simulink model "SB3_subsys_done"  (R2024b)
settings: Solver=FixedStepDiscrete  StartTime=0.0  StopTime=5  FixedStep=0.05  RelTol=1e-3
settings Model: Creator=admin  LastModifiedBy=admin

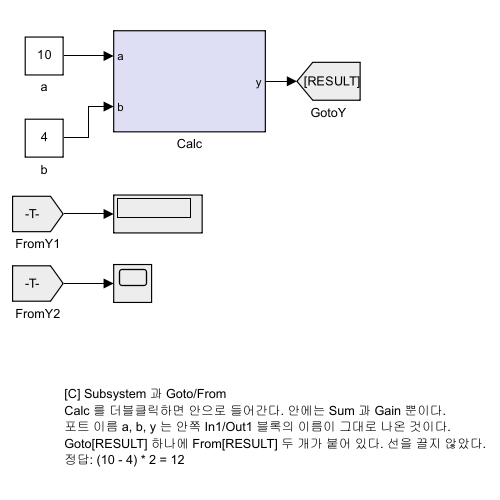
[thumbnail: Simulink's stored preview of the top-level diagram]
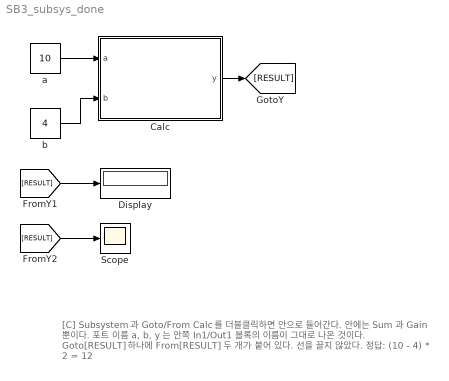
== system SB3_subsys_done ==
  note: [C] Subsystem 과 Goto/From
      | Calc 를 더블클릭하면 안으로 들어간다. 안에는 Sum 과 Gain 뿐이다.
      | 포트 이름 a, b, y 는 안쪽 In1/Out1 블록의 이름이 그대로 나온 것이다.
      | Goto[RESULT] 하나에 From[RESULT] 두 개가 붙어 있다. 선을 끌지 않았다.
      | 정답: (10 - 4) * 2 = 12
  Calc : Subsystem
  Display : Display
  Scope : Scope
  a : Constant  Value=10
  b : Constant  Value=4
  wires:
  a/1 -> Calc/1(a)
  b/1 -> Calc/2(b)
  [RESULT] -> Display/1
  [RESULT] -> Scope/1
  Calc/1(y) -> [RESULT]

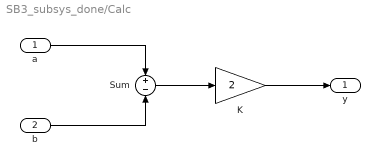
== system SB3_subsys_done/Calc ==
  a : Inport
  b : Inport  Port=2
  K : Gain  Gain=2
  Sum : Sum  Inputs=+-
  y : Outport
  wires:
  a/1 -> Sum/1
  b/1 -> Sum/2
  Sum/1 -> K/1
  K/1 -> y/1
